simulink model "ece456p1"  (R2017b)
settings: Solver=VariableStepAuto  StartTime=0.0  StopTime=20.0  RelTol=1e-3
values from neighbouring files (symbols this model uses):
  kb = .4953    (= 0.4953)    [ece456hw5.m]    (also in ece456hw6.m)
  ke = .3234    (= 0.3234)    [ece456hw5.m]    (also in ece456hw6.m)
  R = 1000    [ece456hw5.m]    (also in ece456hw6.m = 4.67; ece456hw8.m = 0.0721)
  T = 4    [ece456hw5.m]    (also in ece456hw6.m = 0.001; ece456hw8.m = 1.98196948682)
  V = (N.*Y1).*log(X1/IS)    [ece456hw2.m]    (also in ece456hw5.m = 9)
undefined symbols (not defined in the file or in its folder): PW, sigbuilder_block
libraries: powerlib_meascontrol x4
settings Model: Creator=b  LastModifiedBy=b
settings CodeAppCC: StateflowObjectComments=on

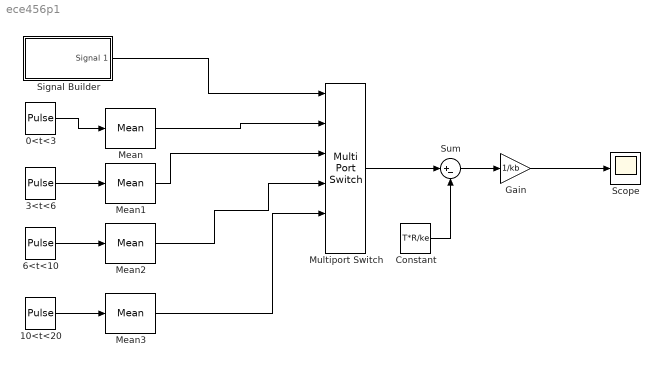
== system ece456p1 ==
  0<t<3 : DiscretePulseGenerator  PulseType=Time based  Amplitude=10  Period=10  PulseWidth=59.58
  10<t<20 : DiscretePulseGenerator  PulseType=Time based  Amplitude=10  Period=10  PulseWidth=PW(4)
  3<t<6 : DiscretePulseGenerator  PulseType=Time based  Amplitude=-10  Period=10  PulseWidth=PW(2)
  6<t<10 : DiscretePulseGenerator  PulseType=Time based  Amplitude=10  Period=10  PulseWidth=PW(3)
  Constant : Constant  Value=T*R/ke
  Gain : Gain  Gain=1/kb
  Mean : powerlib_meascontrol/Measurements/Mean  Freq=1/3  Vinit=V(1)  Ts=0
  Mean1 : powerlib_meascontrol/Measurements/Mean  Freq=1/6  Vinit=V(2)  Ts=0
  Mean2 : powerlib_meascontrol/Measurements/Mean  Freq=1/10  Vinit=V(3)  Ts=0
  Mean3 : powerlib_meascontrol/Measurements/Mean  Freq=1/20  Vinit=V(4)  Ts=0
  Multiport Switch : MultiPortSwitch  Inputs=5
  Scope : Scope
  Signal Builder : Subsystem  Tag=STV Subsys  LoadFcn=sigbuilder_block('load');  StartFcn=sigbuilder_block('start');  StopFcn=sigbuilder_block('stop');  ClipboardFcn=sigbuilder_block('clipboard');  mask(Sigbuilder block){tuvar=[0:10]}
      mask help: Simulink:masks:SigbuilderBlock_MD
      mask init:
      | if ~strcmp(get_param(bdroot(gcbh),'SimulationStatus'),'stopped') tuvar = sigbuilder_block('maskInit'); end
      settings: CopyFcn=sigbuilder_block('copy');  DeleteFcn=sigbuilder_block('delete');  ModelCloseFcn=sigbuilder_block('modelClose');  PreSaveFcn=sigbuilder_block('preSave');  PauseFcn=sigbuilder_block('pause');  ContinueFcn=sigbuilder_block('continue');  NameChangeFcn=sigbuilder_block('namechange');  OpenFcn=sigbuilder_block('open',[362 225 550 400 ]);  CloseFcn=sigbuilder_block('close');
      mask Display: plot(0, 0, 100, 100,[2, 2, 32, 32, 2], [68, 8, 8, 68, 68],[32, 2], [38, 38], [32, 19, 2],[53, 60, 44], [32, 17, 17, 2],[16, 16, 31, 31]);txt = getActiveGroup(gcbh);text(2, 100, txt,'verticalAlignment', 'top');
  Sum : Sum  Inputs=|+-
  wires:
  10<t<20/1 -> Mean3/1
  Signal Builder/1(Signal 1) -> Multiport Switch/1
  6<t<10/1 -> Mean2/1
  Mean/1 -> Multiport Switch/2
  0<t<3/1 -> Mean/1
  Mean1/1 -> Multiport Switch/3
  Mean2/1 -> Multiport Switch/4
  Mean3/1 -> Multiport Switch/5
  3<t<6/1 -> Mean1/1
  Multiport Switch/1 -> Sum/1
  Constant/1 -> Sum/2
  Sum/1 -> Gain/1
  Gain/1 -> Scope/1

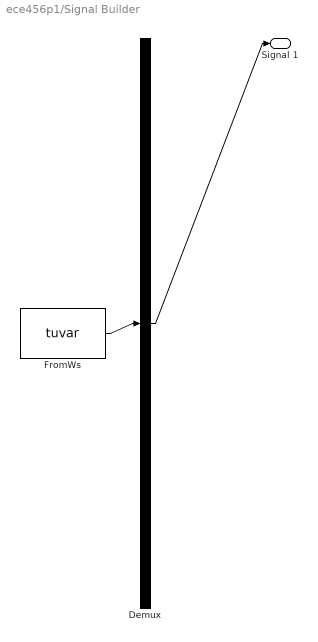
== system ece456p1/Signal Builder ==
  Demux : Demux  Tag=STV Demux  Outputs=1
  FromWs : FromWorkspace  Tag=STV FromWs  VariableName=tuvar  SampleTime=0
      SigBuilderData=|
      | common.afterFinalStr = 'Extrapolate'
      | common.sampleTime = 0
      | dataSet.timeRange = [0 20]
      | dataSet.name = 'Group 1'
      | sbobj.Groups.Name = 'Group 1'
      | sbobj.Groups.Signals.Name = 'Signal 1'
      | sbobj.Groups.Signals.XData = [0 3 3 4 6 6 10 10 20]
      | sbobj.Groups.Signals.YData = [1 1 2 2 2 3 3 4 4]
      | sbobj.Groups.TimeRange = [0 20]
  Signal 1 : Outport  Tag=STV Outport
  wires:
  Demux/1 -> Signal 1/1
  FromWs/1 -> Demux/1
